simulink model "Q2"  (R2020a)
settings: Solver=FixedStepAuto  StartTime=0.0  StopTime=1  FixedStep=1e-6  RelTol=1e-3
libraries: powerlib x10, powerlib_meascontrol x3
settings Model: Creator=seoga  LastModifiedBy=Baris Emektar

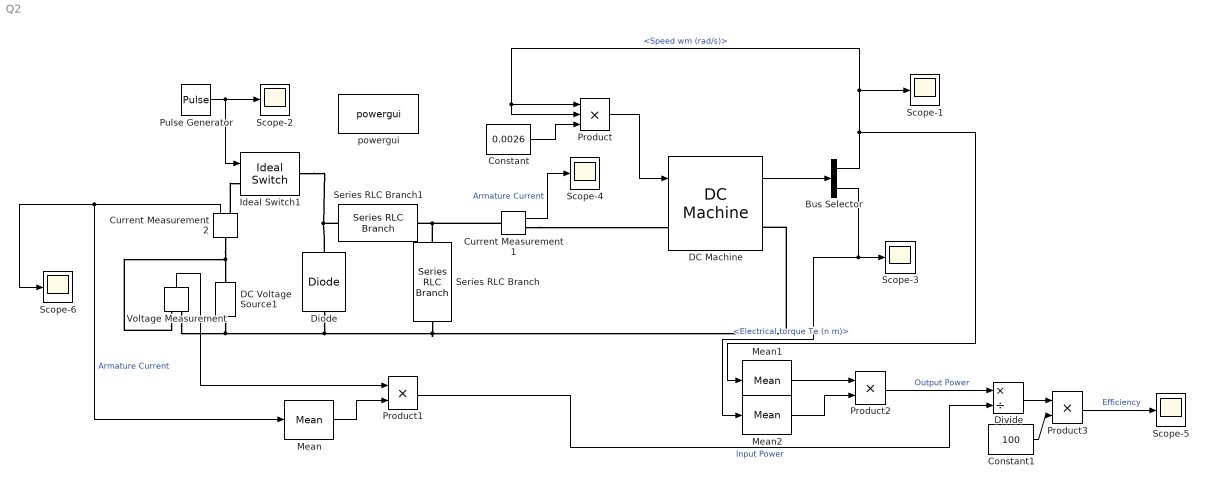
== system Q2 ==
  Bus Selector : BusSelector  OutputSignals=Speed wm (rad/s),Electrical torque Te (n m)
  Constant : Constant  Value=0.0026
  Constant1 : Constant  Value=100
  Current Measurement1 : powerlib/Measurements/Current Measurement  PhasorSimulation=off  OutputType=Complex  PSBequivalent=0
  Current Measurement2 : powerlib/Measurements/Current Measurement  PhasorSimulation=off  OutputType=Complex  PSBequivalent=0
  DC Machine : powerlib/Machines/DC Machine  PresetModel=No  MechanicalLoad=Torque TL  FieldType=Permanent magnet  ShowDetailedParameters=on  MeasurementBus=off  RLa="[ 700e-3  20e-3]"  RLf="[ 240  120]"  Laf=1.8  MachineConstant=Torque constant (N.m/A)  Ke=1.8  Kt=2  J=0.5  Bm=0  Tf=0  w0=1  Ifinit=1  TsPowergui=0  TsBlock=-1
  DC Voltage Source1 : powerlib/Electrical Sources/DC Voltage Source  Amplitude=300  Measurements=None
  Diode : powerlib/Power Electronics/Diode  Ron=0  Lon=0  Vf=0  IC=0  UseSnubber=0  Rs=500  Cs=250e-9  Measurements=off
  Divide : Product  Inputs=*/
  Ideal Switch1 : powerlib/Power Electronics/Ideal Switch  Ron=0  Lon=0  IC=0  Rs=1e5  Cs=inf  Measurements=off
  Mean : powerlib_meascontrol/Measurements/Mean  Freq=100  Vinit=0  Ts=0
  Mean1 : powerlib_meascontrol/Measurements/Mean  Freq=100  Vinit=0  Ts=0
  Mean2 : powerlib_meascontrol/Measurements/Mean  Freq=100  Vinit=0  Ts=0
  Product : Product  Inputs=3
  Product1 : Product
  Product2 : Product
  Product3 : Product
  Pulse Generator : DiscretePulseGenerator  PulseType=Time based  Period=1/25000  PulseWidth=50
  Scope-{1..6} (6 alike) : Scope
  Series RLC Branch : powerlib/Elements/Series RLC Branch  LConnTagsString=__new0  RConnTagsString=__new0  BranchType=C  Resistance=1  Inductance=1e-3  SetiL0=off  InitialCurrent=0  Capacitance=1e-6  Setx0=off  InitialVoltage=0  Measurements=None
  Series RLC Branch1 : powerlib/Elements/Series RLC Branch  LConnTagsString=__new0  RConnTagsString=__new0  BranchType=L  Resistance=1  Inductance=1e-3  SetiL0=off  InitialCurrent=0  Capacitance=1e-6  Setx0=off  InitialVoltage=0  Measurements=None
  Voltage Measurement : powerlib/Measurements/Voltage Measurement  PhasorSimulation=off  OutputType=Complex  PSBequivalent=0
  powergui : powerlib/powergui  Priority=1  SimulationMode=Continuous  SampleTime=50e-6  frequency=60  Iterations=50  frequencyindice=0  Pbase=100e6  ErrMax=1e-4  UnitsV=kV  UnitsW=MW  buscounter=0  FunctionMessages=off  echomessages=off  EnableUseOfTLC=off  CurrentSourceSwitches=off  DisableSnubberDevices=off  DisableRonSwitches=off  DisableVfSwitches=off  DisplayEquations=off  AutomaticDiscreteSolvers=off  SolverType=Tustin/Backward Euler (TBE)  Interpol=off  ExternalGateDelay=off  methode=off  Ts=100  x0status=blocks  SPID=on  SwTol=0  HookPort=off  NonlinearTolerance=1e-4  nMaxIteration=100  ContinueOnMaxIteration=off  RestoreLinks=warning  ResistiveCurrentMeasurement=off  Frange=[0:2:500]  Ylog=off  Xlog=on  ShowGrid=off  save=off  variable=ZData  structure=0  ZoomFFT=off  StartTime=0.0  cycles=1  DisplayStyle=1  fundamental=60  FreqAxis=off  MaxFrequency=1000  frequencyindicesteady=1  RmsSteady=1  display=off
  wires:
  Pulse Generator/1 -> Ideal Switch1/1, Scope-2/1
  Current Measurement1/1 -> Scope-4/1  "Armature Current"
  DC Machine/1 -> Bus Selector/1
  Bus Selector/1 -> Mean1/1, Scope-1/1, Product/1, Product/2  "<Speed wm (rad/s)>"
  Constant/1 -> Product/3
  Product/1 -> DC Machine/1
  Bus Selector/2 -> Scope-3/1, Mean2/1  "<Electrical torque Te (n m)>"
  Current Measurement2/1 -> Scope-6/1, Mean/1  "Armature Current"
  Voltage Measurement/1 -> Product1/1
  Mean/1 -> Product1/2
  Mean2/1 -> Product2/2
  Mean1/1 -> Product2/1
  Product2/1 -> Divide/1  "Output Power"
  Product1/1 -> Divide/2  "Input Power"
  Divide/1 -> Product3/1
  Constant1/1 -> Product3/2
  Product3/1 -> Scope-5/1  "Efficiency"
  connections:
  Current Measurement2/LConn1 -- Voltage Measurement/LConn1 -- DC Voltage Source1/RConn1
  DC Voltage Source1/LConn1 -- Diode/LConn1 -- Series RLC Branch/RConn1 -- DC Machine/RConn1 -- Voltage Measurement/LConn2
  Series RLC Branch1/LConn1 -- Ideal Switch1/RConn1 -- Diode/RConn1
  Current Measurement1/RConn1 -- DC Machine/LConn1
  Current Measurement1/LConn1 -- Series RLC Branch/LConn1 -- Series RLC Branch1/RConn1
  Current Measurement2/RConn1 -- Ideal Switch1/LConn1
